simulink library "WECSim_Lib"  (R2014b)
settings: Solver=ode45  StartTime=0.0  StopTime=10.0  RelTol=1e-3
undefined symbols (not defined in the file): body, constraint, pto, simu, waves, X, Y, Z
libraries: nesl_utility x41, sm_lib x35
(part 1 of 2)
settings Model: Creator=cmichel  LastModifiedBy=cmichel

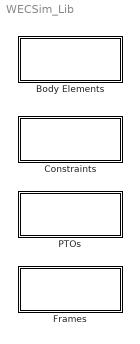
== system WECSim_Lib ==
  Body Elements : Subsystem
      mask Display: text(0,0,' ')
  Constraints : Subsystem
      mask Display: text(0,0,' ')
  Frames : Subsystem
      mask Display: text(0,0,' ')
  PTOs : Subsystem
      mask Display: text(0,0,' ')

== system WECSim_Lib/Body Elements ==
  Rigid Body : Subsystem  mask(BodyElements){body=body(1)}
      mask prompts: body "Body Name:"
      mask help: This block represents a rigid body. The variable name input below must be 'body(i)' where i=1,2,...
      mask init:
      | % Uses:
      | %   body.geometryFile
      | %   body.hydroData.properties.name
      | 
      | if exist('body','var')
      |     h=[gcb '/Structure/Body Properties'];
      |     geomFile=body.geometryFile;
      |     set_param(h,'ExtGeomFileName',geomFile);
      |     h=[gcb '/To Workspace'];
      |     responseName=[body.hydroData.properties.name '_out'];
      |     set_param(h,'VariableName',responseName);
      | end
      | clear bc h geomFile responseName
      settings: AttributesFormatString=%<body>

== system WECSim_Lib/Constraints ==
  Fixed : Subsystem  mask(Constraints){constraint=constraint(1)}
      mask prompts: constraint "Constraint Name:"
      mask help:
      | Does not allow any motion. The variable name input below must be 'constraint(i)' where i=1,2,...
      |
      | constraint(i) must be defined in the input file with the following fields:
      |     .name              = a string
      |     .loc (optional)    = a 3x1 vector [x y z] in m. Default = [0 0 0]
      | The name string is used as the variable name for the output power and as such must comply with all of Matlab's variable naming rules.
      mask init:
      | if exist('constraint','var')
      |     h=[gcb '/output'];
      |     responseName=[constraint.name '_out'];
      |     set_param(h,'VariableName',responseName);
      | end
      | 
      | constraint.checkLoc('W');
      settings: AttributesFormatString=%<constraint>
  Floating : Subsystem  mask(Constraints){constraint=constraint(1)}
      mask prompts: constraint "Constraint Name:"
      mask help:
      | Allows body to be free floating (motion in Surge, Heave, and Pitch). The variable name input below must be 'constraint(i)' where i=1,2,...
      |
      | constraint(i) must be defined in the input file with the following fields:
      |     .name              = a string
      |     .loc (optional)    = a 3x1 vector [x y z] in m. Default = [0 0 0]
      |
      | The name string is used as the variable name for the output power and as such must comply with all of Matlab's variable naming rules.
      mask init:
      | if exist('constraint','var')
      |     h=[gcb '/output'];
      |     responseName=[constraint.name '_out'];
      |     set_param(h,'VariableName',responseName);
      | end
      | 
      | constraint.checkLoc('W');
      settings: AttributesFormatString=%<constraint>
  Heave : Subsystem  mask(Constraints){constraint=constraint(1)}
      mask prompts: constraint "Constraint Name:"
      mask help:
      | Constrains motion to Heave translation only.The variable name input below must be 'constraint(i)' where i=1,2,...
      |
      | constraint(i) must be defined in the input file with the following fields:
      |     .name              = a string
      |     .loc (optional)    = a 3x1 vector [x y z] in m. Default = [0 0 0]
      | The name string is used as the variable name for the output power and as such must comply with all of Matlab's variable naming rules.
      mask init:
      | if exist('constraint','var')
      |     h=[gcb '/output'];
      |     responseName=[constraint.name '_out'];
      |     set_param(h,'VariableName',responseName);
      | end
      | 
      | constraint.checkLoc('W');
      settings: AttributesFormatString=%<constraint>
  Pitch : Subsystem  mask(Constraints){constraint=constraint(1)}
      mask prompts: constraint "Constraint Name:"
      mask help:
      | Constrains motion to Pitch rotation only. The variable name input below must be 'constraint(i)' where i=1,2,...
      |
      | constraint(i) must be defined in the input file with the following fields:
      |     .name   = a string
      |     .loc    = a 3x1 vector [x y z] in m
      |
      | The name string is used as the variable name for the output power and as such must comply with all of Matlab's variable naming rules.
      mask init:
      | if exist('constraint','var')
      |     h=[gcb '/output'];
      |     responseName=[constraint.name '_out'];
      |     set_param(h,'VariableName',responseName);
      | end
      | 
      | constraint.checkLoc('E');
      settings: AttributesFormatString=%<constraint>
  Surge : Subsystem  mask(Constraints){constraint=constraint(1)}
      mask prompts: constraint "Constraint Name:"
      mask help:
      | Constrains motion to Surge translation only.The variable name input below must be 'constraint(i)' where i=1,2,...
      |
      | constraint(i) must be defined in the input file with the following fields:
      |     .name              = a string
      |     .loc (optional)    = a 3x1 vector [x y z] in m. Default = [0 0 0]
      |
      | The name string is used as the variable name for the output power and as such must comply with all of Matlab's variable naming rules.
      mask init:
      | if exist('constraint','var')
      |     h=[gcb '/output'];
      |     responseName=[constraint.name '_out'];
      |     set_param(h,'VariableName',responseName);
      | end
      | 
      | constraint.checkLoc('W');
      settings: AttributesFormatString=%<constraint>

== system WECSim_Lib/Frames ==
  Global Reference Frame : Subsystem  mask(Frames){waves=waves, simu=simu}
      mask prompts: waves "Wave Class Name"; simu "Simulation Class Name"
      mask help:
      | This block contains Global References, including solver configurations, free surface and seabed description, and simulation time.
      | It uses the following fields from the Simulation and Wave classes:
      |
      | Simulation Class:
      |     .endTime
      |     .dt
      |     .domainSize
      |
      | Wave Class:
      |     .waterDepth

== system WECSim_Lib/PTOs ==
  Rotational PTO (Local RY) : Subsystem  mask(PTO){pto=pto(1)}
      mask prompts: pto "PTO Name:"
      mask help:
      | This PTO constrains the follower (F) to only rotate about the Y-axis of the base (B), and applies a PTO stiffness and damping value. The variable name input below must be 'pto(i)' where i=1,2,...
      |
      | pto(i) must be defined in the input file with the following fields:
      |     .name   = a string
      |     .k      = a scalar in N*m/radians
      |     .c      = a scalar in N*m/(radians/s)
      |     .loc    = a 3x1 vector [x y z] in m
      |
      | The name string is used as the variable name for the output power and as such must comply with all of Matlab's variable naming rules.
      mask init:
      | if exist('pto','var')
      |     h=[gcb '/output'];
      |     responseName=[pto.name '_out'];
      |     set_param(h,'VariableName',responseName);
      | end
      | 
      | pto.checkLoc('E');
      settings: AttributesFormatString=%<pto>
  Translational PTO (Local X) : Subsystem  mask(PTO){pto=pto(1)}
      mask prompts: pto "PTO Name:"
      mask help:
      | This PTO constrains the follower (F) to only move along the X-direction of the base (B), and applies a PTO stiffness and damping value. The variable name input below must be 'pto(i)' where i=1,2,...
      |
      | pto(i) must be defined in the input file with the following fields:
      |     .name              = a string
      |     .k                 = a scalar in N/m
      |     .c                 = a scalar in N/(m/s)
      |     .loc (optional)    = a 3x1 vector [x y z] in m. Default = [0 0 0]
      | The name string is used as the variable name for the output power and as such must comply with all of Matlab's variable naming rules.
      mask init:
      | if exist('pto','var')
      |     h=[gcb '/output'];
      |     responseName=[pto.name '_out'];
      |     set_param(h,'VariableName',responseName);
      | end
      | 
      | pto.checkLoc('W');
      settings: AttributesFormatString=%<pto>
  Translational PTO (Local Z) : Subsystem  mask(PTO){pto=pto(1)}
      mask prompts: pto "PTO Name:"
      mask help:
      | This PTO constrains the follower (F) to only move along the Z-direction of the base (B), and applies a PTO stiffness and damping value. The variable name input below must be 'pto(i)' where i=1,2,...
      |
      | pto(i) must be defined in the input file with the following fields:
      |     .name               = a string
      |     .k                  = a scalar in N/m
      |     .c                  = a scalar in N/(m/s)
      |     .loc (optional)     = a 3x1 vector [x y z] in m. Default = [0 0 0]
      |
      | The name string is used as the variable name for the output power and as such must comply with all of Matlab's variable naming rules.
      mask init:
      | if exist('pto','var')
      |     h=[gcb '/output'];
      |     responseName=[pto.name '_out'];
      |     set_param(h,'VariableName',responseName);
      | end
      | 
      | pto.checkLoc('W');
      settings: AttributesFormatString=%<pto>

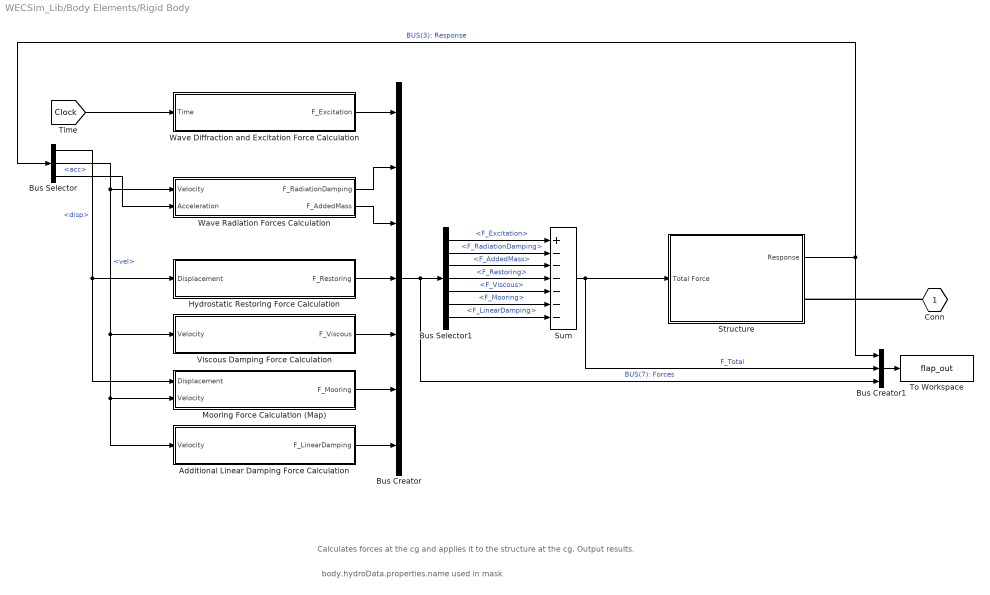
== system WECSim_Lib/Body Elements/Rigid Body ==
  note: body.hydroData.properties.name used in mask
  note: Calculates forces at the cg and applies it to the structure at the cg. Output results.
  Additional Linear Damping Force Calculation : Subsystem
  Bus Creator : BusCreator  Inputs=7
  Bus Creator1 : BusCreator  Inputs=3
  Bus Selector : BusSelector  OutputSignals=disp,vel,acc
  Bus Selector1 : BusSelector  OutputSignals=F_Excitation,F_RadiationDamping,F_AddedMass,F_Restoring,F_Viscous,F_Mooring,F_LinearDamping
  Hydrostatic Restoring Force Calculation : Subsystem
  Mooring Force Calculation (Map) : Subsystem
  Structure : Subsystem
  Sum : Sum  Inputs=+------
  To Workspace : ToWorkspace  VariableName=flap_out  SaveFormat=Structure With Time  SampleTime=-1
  Viscous Damping Force Calculation : Subsystem
  Wave Diffraction and Excitation Force Calculation : Subsystem
  Wave Radiation Forces Calculation : Subsystem
  Conn : PMIOPort  Port=1  Side=Right
  wires:
  Sum/1 -> Bus Creator1/2, Structure/1(Total Force)  "F_Total"
  Bus Selector/1 -> Mooring Force Calculation (Map)/1(Displacement), Hydrostatic Restoring Force Calculation/1(Displacement)  "<disp>"
  Structure/1(Response) -> Bus Creator1/1, Bus Selector/1  "BUS(3): Response"
  Bus Creator/1 -> Bus Creator1/3, Bus Selector1/1  "BUS(7): Forces"
  Bus Creator1/1 -> To Workspace/1
  Mooring Force Calculation (Map)/1(F_Mooring) -> Bus Creator/6
  Viscous Damping Force Calculation/1(F_Viscous) -> Bus Creator/5
  Hydrostatic Restoring Force Calculation/1(F_Restoring) -> Bus Creator/4
  Wave Radiation Forces Calculation/1(F_RadiationDamping) -> Bus Creator/2
  Wave Diffraction and Excitation Force Calculation/1(F_Excitation) -> Bus Creator/1
  Additional Linear Damping Force Calculation/1(F_LinearDamping) -> Bus Creator/7
  Bus Selector/2 -> Additional Linear Damping Force Calculation/1(Velocity), Mooring Force Calculation (Map)/2(Velocity), Viscous Damping Force Calculation/1(Velocity), Wave Radiation Forces Calculation/1(Velocity)  "<vel>"
  Bus Selector/3 -> Wave Radiation Forces Calculation/2(Acceleration)  "<acc>"
  Wave Radiation Forces Calculation/2(F_AddedMass) -> Bus Creator/3
  Bus Selector1/4 -> Sum/4  "<F_Restoring>"
  Bus Selector1/3 -> Sum/3  "<F_AddedMass>"
  Bus Selector1/5 -> Sum/5  "<F_Viscous>"
  Bus Selector1/2 -> Sum/2  "<F_RadiationDamping>"
  Bus Selector1/6 -> Sum/6  "<F_Mooring>"
  Bus Selector1/1 -> Sum/1  "<F_Excitation>"
  Bus Selector1/7 -> Sum/7  "<F_LinearDamping>"
  [Clock] -> Wave Diffraction and Excitation Force Calculation/1(Time)
  connections:
  Conn/RConn1 -- Structure/RConn1

== system WECSim_Lib/Constraints/Fixed ==
  note: constraint.loc
      | constraint.c
      | constraint.k
      | constraint.name used in mask
  note: Constraints the motion to the desired DOF.
      | Moves the connection points (B and F) from the free surface to the PTO location.
      | Outputs forces and motions.
  Mux : Mux  Inputs=2
  PS-Simulink Converter : nesl_utility/PS-Simulink Converter  PhysicalDomain=network_engine_domain  SubClassName=ps_output  LeftPortType=input  RightPortType=output  PseudoPeriodic=off  Frequencies=[]  Unit=1  AffineConversion=off
  PS-Simulink Converter1 : nesl_utility/PS-Simulink Converter  PhysicalDomain=network_engine_domain  SubClassName=ps_output  LeftPortType=input  RightPortType=output  PseudoPeriodic=off  Frequencies=[]  Unit=1  AffineConversion=off
  Rigid Transform : sm_lib/Frames and Transforms/Rigid Transform  TranslationMethod=Cartesian  TranslationLengthUnit=m  TranslationStandardAxis=+Z  TranslationStandardOffset=0  TranslationCartesianOffset=constraint.loc  TranslationROffset=0  TranslationROffsetUnits=m  TranslationZOffset=0  TranslationZOffsetUnits=m  TranslationThetaOffset=0  TranslationThetaOffsetUnits=deg  RotationMethod=None  RotationAngleUnits=deg  RotationStandardAxis=+X  RotationAngle=90  RotationArbitraryAxis=[0 0 1]  FollAlignAxisA=+X  BaseAlignAxisA=+Y  FollAlignAxisB=+Y  BaseAlignAxisB=+Z  RotationMatrix=[1 0 0; 0 1 0; 0 0 1]  BlockFunction=simmechanics.library.frames_transforms.rigid_transform
  Rigid Transform1 : sm_lib/Frames and Transforms/Rigid Transform  TranslationMethod=Cartesian  TranslationLengthUnit=m  TranslationStandardAxis=+Z  TranslationStandardOffset=0  TranslationCartesianOffset=constraint.loc  TranslationROffset=0  TranslationROffsetUnits=m  TranslationZOffset=0  TranslationZOffsetUnits=m  TranslationThetaOffset=0  TranslationThetaOffsetUnits=deg  RotationMethod=None  RotationAngleUnits=deg  RotationStandardAxis=+X  RotationAngle=90  RotationArbitraryAxis=[0 0 1]  FollAlignAxisA=+X  BaseAlignAxisA=+Y  FollAlignAxisB=+Y  BaseAlignAxisB=+Z  RotationMatrix=[1 0 0; 0 1 0; 0 0 1]  BlockFunction=simmechanics.library.frames_transforms.rigid_transform
  Weld Joint (Fixed) : sm_lib/Joints/Weld Joint  SenseConstraintForce=on  SenseConstraintForceX=off  SenseConstraintForceY=off  SenseConstraintForceZ=off  SenseConstraintTorque=on  SenseConstraintTorqueX=off  SenseConstraintTorqueY=off  SenseConstraintTorqueZ=off  SenseTotalForce=off  SenseTotalForceX=off  SenseTotalForceY=off  SenseTotalForceZ=off  SenseTotalTorque=off  SenseTotalTorqueX=off  SenseTotalTorqueY=off  SenseTotalTorqueZ=off  CompositeWrenchDir=BaseOnFollower  CompositeWrenchFrame=BaseFrame  BlockFunction=simmechanics.library.joints.weld_joint
  output : ToWorkspace  VariableName=Constraint1_out  SaveFormat=Structure With Time  SampleTime=-1
  B : PMIOPort  Port=1  Side=Left
  F : PMIOPort  Port=2  Side=Right
  wires:
  PS-Simulink Converter/1 -> Mux/1
  PS-Simulink Converter1/1 -> Mux/2
  Mux/1 -> output/1  "Constraint Forces"
  connections:
  PS-Simulink Converter1/LConn1 -- Weld Joint (Fixed)/RConn3
  PS-Simulink Converter/LConn1 -- Weld Joint (Fixed)/RConn2
  F/RConn1 -- Rigid Transform1/LConn1
  Rigid Transform1/RConn1 -- Weld Joint (Fixed)/RConn1
  Weld Joint (Fixed)/LConn1 -- Rigid Transform/RConn1
  Rigid Transform/LConn1 -- B/RConn1

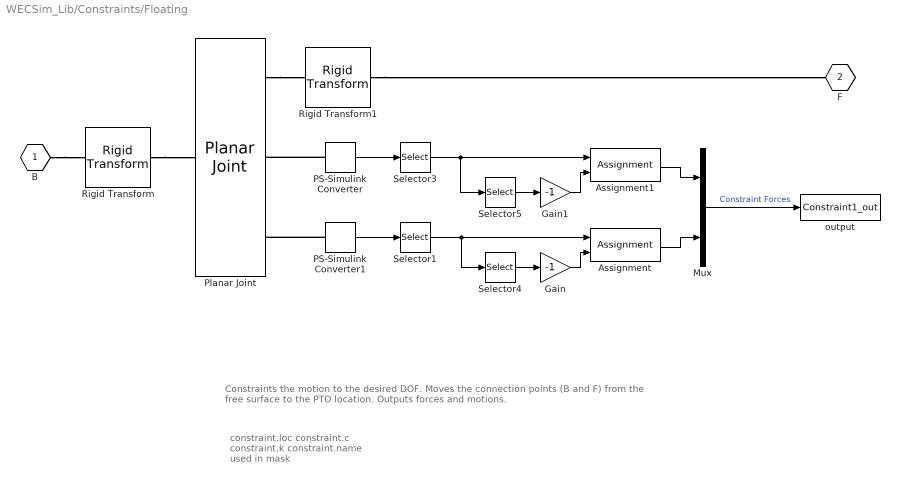
== system WECSim_Lib/Constraints/Floating ==
  note: constraint.loc
      | constraint.c
      | constraint.k
      | constraint.name used in mask
  note: Constraints the motion to the desired DOF.
      | Moves the connection points (B and F) from the free surface to the PTO location.
      | Outputs forces and motions.
  Assignment : Assignment  DiagnosticForDimensions=Warning  Indices=2
  Assignment1 : Assignment  DiagnosticForDimensions=Warning  Indices=2
  Gain : Gain  Gain=-1
  Gain1 : Gain  Gain=-1
  Mux : Mux  Inputs=2
  PS-Simulink Converter : nesl_utility/PS-Simulink Converter  PhysicalDomain=network_engine_domain  SubClassName=ps_output  LeftPortType=input  RightPortType=output  PseudoPeriodic=off  Frequencies=[]  Unit=1  AffineConversion=off
  PS-Simulink Converter1 : nesl_utility/PS-Simulink Converter  PhysicalDomain=network_engine_domain  SubClassName=ps_output  LeftPortType=input  RightPortType=output  PseudoPeriodic=off  Frequencies=[]  Unit=1  AffineConversion=off
  Planar Joint : sm_lib/Joints/Planar Joint  SenseConstraintForce=on  SenseConstraintForceX=off  SenseConstraintForceY=off  SenseConstraintForceZ=off  SenseConstraintTorque=on  SenseConstraintTorqueX=off  SenseConstraintTorqueY=off  SenseConstraintTorqueZ=off  SenseTotalForce=off  SenseTotalForceX=off  SenseTotalForceY=off  SenseTotalForceZ=off  SenseTotalTorque=off  SenseTotalTorqueX=off  SenseTotalTorqueY=off  SenseTotalTorqueZ=off  CompositeWrenchDir=BaseOnFollower  CompositeWrenchFrame=BaseFrame  PxEquilibriumPosition=0  PxEquilibriumPositionUnits=m  PxSpringStiffness=0  PxSpringStiffnessUnits=N/m  PxDampingCoefficient=0  PxDampingCoefficientUnits=N/(m/s)  PxTorqueActuationMode=NoTorque  PxMotionActuationMode=ComputedMotion  PxSensePosition=off  PxSenseVelocity=off  PxSenseAcceleration=off  PxSenseTorqueForce=off  PxPositionTargetValue=0  PxPositionTargetValueUnits=m  PxPositionTargetSpecify=off  PxPositionTargetPriority=High  PxVelocityTargetValue=0  PxVelocityTargetValueUnits=m/s  PxVelocityTargetSpecify=off  PxVelocityTargetPriority=High  PyEquilibriumPosition=0  PyEquilibriumPositionUnits=m  PySpringStiffness=0  PySpringStiffnessUnits=N/m  PyDampingCoefficient=0  PyDampingCoefficientUnits=N/(m/s)  PyTorqueActuationMode=NoTorque  PyMotionActuationMode=ComputedMotion  PySensePosition=off  PySenseVelocity=off  PySenseAcceleration=off  PySenseTorqueForce=off  PyPositionTargetValue=0  PyPositionTargetValueUnits=m  PyPositionTargetSpecify=off  PyPositionTargetPriority=High  PyVelocityTargetValue=0  PyVelocityTargetValueUnits=m/s  PyVelocityTargetSpecify=off  PyVelocityTargetPriority=High  RzEquilibriumPosition=0  RzEquilibriumPositionUnits=deg  RzSpringStiffness=0  RzSpringStiffnessUnits=N*m/deg  RzDampingCoefficient=0  RzDampingCoefficientUnits=N*m/(deg/s)  RzTorqueActuationMode=NoTorque  RzMotionActuationMode=ComputedMotion  RzSensePosition=off  RzSenseVelocity=off  RzSenseAcceleration=off  RzSenseTorqueForce=off  RzPositionTargetValue=0  RzPositionTargetValueUnits=deg  RzPositionTargetSpecify=off  RzPositionTargetPriority=High  RzVelocityTargetValue=0  RzVelocityTargetValueUnits=deg/s  RzVelocityTargetSpecify=off  RzVelocityTargetPriority=High  BlockFunction=simmechanics.library.joints.planar_joint
  Rigid Transform : sm_lib/Frames and Transforms/Rigid Transform  TranslationMethod=Cartesian  TranslationLengthUnit=m  TranslationStandardAxis=+Z  TranslationStandardOffset=0  TranslationCartesianOffset=constraint.loc  TranslationROffset=0  TranslationROffsetUnits=m  TranslationZOffset=0  TranslationZOffsetUnits=m  TranslationThetaOffset=0  TranslationThetaOffsetUnits=deg  RotationMethod=StandardAxis  RotationAngleUnits=deg  RotationStandardAxis=+X  RotationAngle=90  RotationArbitraryAxis=[0 0 1]  FollAlignAxisA=+X  BaseAlignAxisA=+Y  FollAlignAxisB=+Y  BaseAlignAxisB=+Z  RotationMatrix=[1 0 0; 0 1 0; 0 0 1]  BlockFunction=simmechanics.library.frames_transforms.rigid_transform
  Rigid Transform1 : sm_lib/Frames and Transforms/Rigid Transform  TranslationMethod=Cartesian  TranslationLengthUnit=m  TranslationStandardAxis=+Z  TranslationStandardOffset=0  TranslationCartesianOffset=constraint.loc  TranslationROffset=0  TranslationROffsetUnits=m  TranslationZOffset=0  TranslationZOffsetUnits=m  TranslationThetaOffset=0  TranslationThetaOffsetUnits=deg  RotationMethod=StandardAxis  RotationAngleUnits=deg  RotationStandardAxis=+X  RotationAngle=90  RotationArbitraryAxis=[0 0 1]  FollAlignAxisA=+X  BaseAlignAxisA=+Y  FollAlignAxisB=+Y  BaseAlignAxisB=+Z  RotationMatrix=[1 0 0; 0 1 0; 0 0 1]  BlockFunction=simmechanics.library.frames_transforms.rigid_transform
  Selector1 : Selector  InputPortWidth=3  Indices=[1 3 2]
  Selector3 : Selector  InputPortWidth=3  Indices=[1 3 2]
  Selector4 : Selector  InputPortWidth=3  Indices=[2]
  Selector5 : Selector  InputPortWidth=3  Indices=[2]
  output : ToWorkspace  VariableName=Constraint1_out  SaveFormat=Structure With Time  SampleTime=-1
  B : PMIOPort  Port=1  Side=Left
  F : PMIOPort  Port=2  Side=Right
  wires:
  Mux/1 -> output/1  "Constraint Forces"
  Selector1/1 -> Assignment/1, Selector4/1
  Selector4/1 -> Gain/1
  Gain/1 -> Assignment/2
  Selector3/1 -> Assignment1/1, Selector5/1
  Selector5/1 -> Gain1/1
  Gain1/1 -> Assignment1/2
  PS-Simulink Converter1/1 -> Selector1/1
  PS-Simulink Converter/1 -> Selector3/1
  Assignment/1 -> Mux/2
  Assignment1/1 -> Mux/1
  connections:
  Rigid Transform1/LConn1 -- F/RConn1
  Planar Joint/RConn1 -- Rigid Transform1/RConn1
  Rigid Transform/RConn1 -- Planar Joint/LConn1
  B/RConn1 -- Rigid Transform/LConn1
  PS-Simulink Converter/LConn1 -- Planar Joint/RConn2
  PS-Simulink Converter1/LConn1 -- Planar Joint/RConn3

== system WECSim_Lib/Constraints/Heave ==
  note: constraint.loc
      | constraint.c
      | constraint.k
      | constraint.name used in mask
  note: Constraints the motion to the desired DOF.
      | Moves the connection points (B and F) from the free surface to the PTO location.
      | Outputs forces and motions.
  Mux : Mux  Inputs=2
  PS-Simulink Converter : nesl_utility/PS-Simulink Converter  PhysicalDomain=network_engine_domain  SubClassName=ps_output  LeftPortType=input  RightPortType=output  PseudoPeriodic=off  Frequencies=[]  Unit=1  AffineConversion=off
  PS-Simulink Converter1 : nesl_utility/PS-Simulink Converter  PhysicalDomain=network_engine_domain  SubClassName=ps_output  LeftPortType=input  RightPortType=output  PseudoPeriodic=off  Frequencies=[]  Unit=1  AffineConversion=off
  Prismatic Joint (Translational Constraint) : sm_lib/Joints/Prismatic Joint  SenseConstraintForce=on  SenseConstraintForceX=off  SenseConstraintForceY=off  SenseConstraintForceZ=off  SenseConstraintTorque=on  SenseConstraintTorqueX=off  SenseConstraintTorqueY=off  SenseConstraintTorqueZ=off  SenseTotalForce=off  SenseTotalForceX=off  SenseTotalForceY=off  SenseTotalForceZ=off  SenseTotalTorque=off  SenseTotalTorqueX=off  SenseTotalTorqueY=off  SenseTotalTorqueZ=off  CompositeWrenchDir=BaseOnFollower  CompositeWrenchFrame=BaseFrame  EquilibriumPosition=0  EquilibriumPositionUnits=m  SpringStiffness=0  SpringStiffnessUnits=N/m  DampingCoefficient=0  DampingCoefficientUnits=N/(m/s)  TorqueActuationMode=NoTorque  MotionActuationMode=ComputedMotion  SensePosition=off  SenseVelocity=off  SenseAcceleration=off  SenseTorqueForce=off  PositionTargetValue=0  PositionTargetValueUnits=m  PositionTargetSpecify=off  PositionTargetPriority=High  VelocityTargetValue=0  VelocityTargetValueUnits=m/s  VelocityTargetSpecify=off  VelocityTargetPriority=High  BlockFunction=simmechanics.library.joints.prismatic_joint
  Rigid Transform : sm_lib/Frames and Transforms/Rigid Transform  TranslationMethod=Cartesian  TranslationLengthUnit=m  TranslationStandardAxis=+Z  TranslationStandardOffset=0  TranslationCartesianOffset=constraint.loc  TranslationROffset=0  TranslationROffsetUnits=m  TranslationZOffset=0  TranslationZOffsetUnits=m  TranslationThetaOffset=0  TranslationThetaOffsetUnits=deg  RotationMethod=None  RotationAngleUnits=deg  RotationStandardAxis=+X  RotationAngle=90  RotationArbitraryAxis=[0 0 1]  FollAlignAxisA=+X  BaseAlignAxisA=+Y  FollAlignAxisB=+Y  BaseAlignAxisB=+Z  RotationMatrix=[1 0 0; 0 1 0; 0 0 1]  BlockFunction=simmechanics.library.frames_transforms.rigid_transform
  Rigid Transform1 : sm_lib/Frames and Transforms/Rigid Transform  TranslationMethod=Cartesian  TranslationLengthUnit=m  TranslationStandardAxis=+Z  TranslationStandardOffset=0  TranslationCartesianOffset=constraint.loc  TranslationROffset=0  TranslationROffsetUnits=m  TranslationZOffset=0  TranslationZOffsetUnits=m  TranslationThetaOffset=0  TranslationThetaOffsetUnits=deg  RotationMethod=None  RotationAngleUnits=deg  RotationStandardAxis=+X  RotationAngle=90  RotationArbitraryAxis=[0 0 1]  FollAlignAxisA=+X  BaseAlignAxisA=+Y  FollAlignAxisB=+Y  BaseAlignAxisB=+Z  RotationMatrix=[1 0 0; 0 1 0; 0 0 1]  BlockFunction=simmechanics.library.frames_transforms.rigid_transform
  output : ToWorkspace  VariableName=Constraint1_out  SaveFormat=Structure With Time  SampleTime=-1
  F : PMIOPort  Port=1  Side=Right
  B : PMIOPort  Port=2  Side=Left
  wires:
  PS-Simulink Converter/1 -> Mux/1
  PS-Simulink Converter1/1 -> Mux/2
  Mux/1 -> output/1  "Constraint Forces"
  connections:
  PS-Simulink Converter/LConn1 -- Prismatic Joint (Translational Constraint)/RConn2
  PS-Simulink Converter1/LConn1 -- Prismatic Joint (Translational Constraint)/RConn3
  Rigid Transform1/RConn1 -- Prismatic Joint (Translational Constraint)/RConn1
  Rigid Transform1/LConn1 -- F/RConn1
  B/RConn1 -- Rigid Transform/LConn1
  Rigid Transform/RConn1 -- Prismatic Joint (Translational Constraint)/LConn1

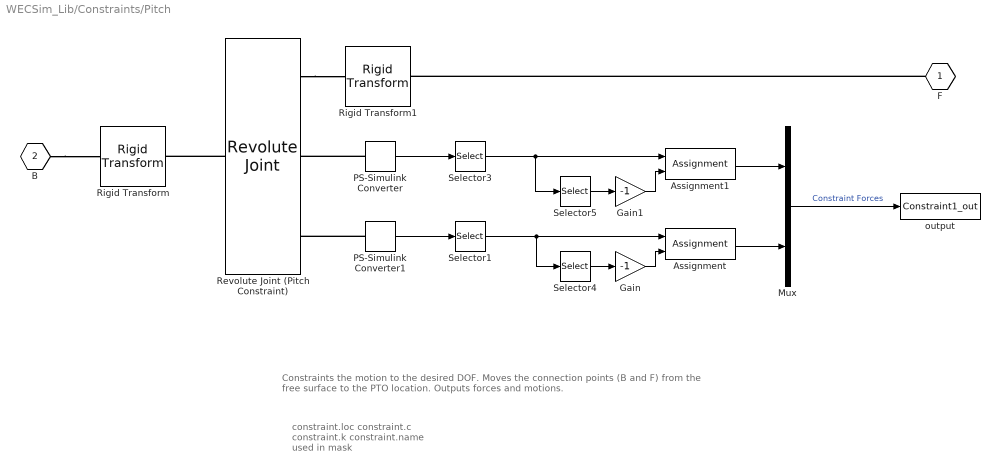
== system WECSim_Lib/Constraints/Pitch ==
  note: constraint.loc
      | constraint.c
      | constraint.k
      | constraint.name used in mask
  note: Constraints the motion to the desired DOF.
      | Moves the connection points (B and F) from the free surface to the PTO location.
      | Outputs forces and motions.
  Assignment : Assignment  DiagnosticForDimensions=Warning  Indices=2
  Assignment1 : Assignment  DiagnosticForDimensions=Warning  Indices=2
  Gain : Gain  Gain=-1
  Gain1 : Gain  Gain=-1
  Mux : Mux  Inputs=2
  PS-Simulink Converter : nesl_utility/PS-Simulink Converter  PhysicalDomain=network_engine_domain  SubClassName=ps_output  LeftPortType=input  RightPortType=output  PseudoPeriodic=off  Frequencies=[]  Unit=1  AffineConversion=off
  PS-Simulink Converter1 : nesl_utility/PS-Simulink Converter  PhysicalDomain=network_engine_domain  SubClassName=ps_output  LeftPortType=input  RightPortType=output  PseudoPeriodic=off  Frequencies=[]  Unit=1  AffineConversion=off
  Revolute Joint (Pitch Constraint) : sm_lib/Joints/Revolute Joint  SenseConstraintForce=on  SenseConstraintForceX=off  SenseConstraintForceY=off  SenseConstraintForceZ=off  SenseConstraintTorque=on  SenseConstraintTorqueX=off  SenseConstraintTorqueY=off  SenseConstraintTorqueZ=off  SenseTotalForce=off  SenseTotalForceX=off  SenseTotalForceY=off  SenseTotalForceZ=off  SenseTotalTorque=off  SenseTotalTorqueX=off  SenseTotalTorqueY=off  SenseTotalTorqueZ=off  CompositeWrenchDir=BaseOnFollower  CompositeWrenchFrame=BaseFrame  EquilibriumPosition=0  EquilibriumPositionUnits=deg  SpringStiffness=0  SpringStiffnessUnits=N*m/deg  DampingCoefficient=0  DampingCoefficientUnits=N*m/(rad/s)  TorqueActuationMode=NoTorque  MotionActuationMode=ComputedMotion  SensePosition=off  SenseVelocity=off  SenseAcceleration=off  SenseTorqueForce=off  PositionTargetValue=0  PositionTargetValueUnits=deg  PositionTargetSpecify=off  PositionTargetPriority=High  VelocityTargetValue=0  VelocityTargetValueUnits=deg/s  VelocityTargetSpecify=off  VelocityTargetPriority=High  BlockFunction=simmechanics.library.joints.revolute_joint
  Rigid Transform : sm_lib/Frames and Transforms/Rigid Transform  TranslationMethod=Cartesian  TranslationLengthUnit=m  TranslationStandardAxis=+Z  TranslationStandardOffset=0  TranslationCartesianOffset=constraint.loc  TranslationROffset=0  TranslationROffsetUnits=m  TranslationZOffset=0  TranslationZOffsetUnits=m  TranslationThetaOffset=0  TranslationThetaOffsetUnits=deg  RotationMethod=StandardAxis  RotationAngleUnits=deg  RotationStandardAxis=+X  RotationAngle=90  RotationArbitraryAxis=[0 0 1]  FollAlignAxisA=+X  BaseAlignAxisA=+Y  FollAlignAxisB=+Y  BaseAlignAxisB=+Z  RotationMatrix=[1 0 0; 0 1 0; 0 0 1]  BlockFunction=simmechanics.library.frames_transforms.rigid_transform
  Rigid Transform1 : sm_lib/Frames and Transforms/Rigid Transform  TranslationMethod=Cartesian  TranslationLengthUnit=m  TranslationStandardAxis=+Z  TranslationStandardOffset=0  TranslationCartesianOffset=constraint.loc  TranslationROffset=0  TranslationROffsetUnits=m  TranslationZOffset=0  TranslationZOffsetUnits=m  TranslationThetaOffset=0  TranslationThetaOffsetUnits=deg  RotationMethod=StandardAxis  RotationAngleUnits=deg  RotationStandardAxis=+X  RotationAngle=90  RotationArbitraryAxis=[0 0 1]  FollAlignAxisA=+X  BaseAlignAxisA=+Y  FollAlignAxisB=+Y  BaseAlignAxisB=+Z  RotationMatrix=[1 0 0; 0 1 0; 0 0 1]  BlockFunction=simmechanics.library.frames_transforms.rigid_transform
  Selector1 : Selector  InputPortWidth=3  Indices=[1 3 2]
  Selector3 : Selector  InputPortWidth=3  Indices=[1 3 2]
  Selector4 : Selector  InputPortWidth=3  Indices=[2]
  Selector5 : Selector  InputPortWidth=3  Indices=[2]
  output : ToWorkspace  VariableName=Constraint1_out  SaveFormat=Structure With Time  SampleTime=-1
  F : PMIOPort  Port=1  Side=Right
  B : PMIOPort  Port=2  Side=Left
  wires:
  Mux/1 -> output/1  "Constraint Forces"
  PS-Simulink Converter/1 -> Selector3/1
  PS-Simulink Converter1/1 -> Selector1/1
  Selector1/1 -> Selector4/1, Assignment/1
  Selector4/1 -> Gain/1
  Gain/1 -> Assignment/2
  Assignment/1 -> Mux/2
  Selector3/1 -> Selector5/1, Assignment1/1
  Selector5/1 -> Gain1/1
  Gain1/1 -> Assignment1/2
  Assignment1/1 -> Mux/1
  connections:
  Revolute Joint (Pitch Constraint)/LConn1 -- Rigid Transform/RConn1
  Revolute Joint (Pitch Constraint)/RConn1 -- Rigid Transform1/RConn1
  B/RConn1 -- Rigid Transform/LConn1
  F/RConn1 -- Rigid Transform1/LConn1
  PS-Simulink Converter/LConn1 -- Revolute Joint (Pitch Constraint)/RConn2
  PS-Simulink Converter1/LConn1 -- Revolute Joint (Pitch Constraint)/RConn3

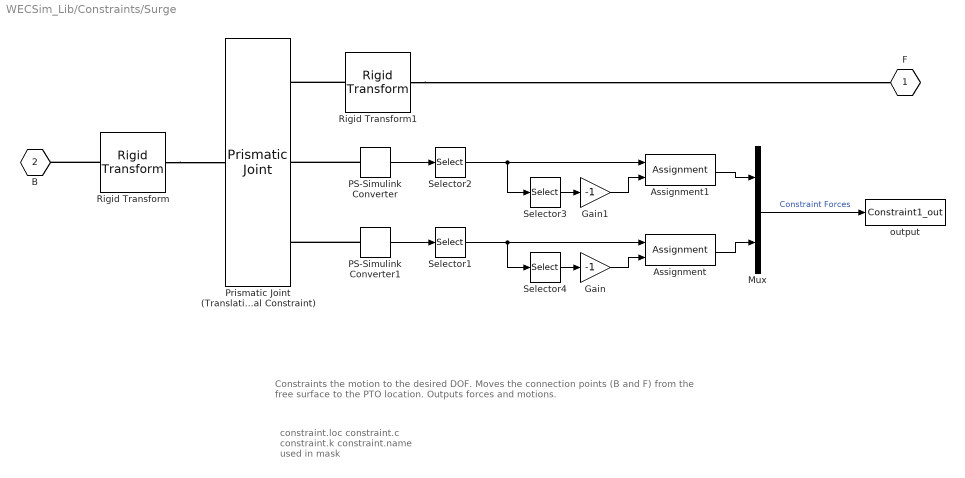
== system WECSim_Lib/Constraints/Surge ==
  note: constraint.loc
      | constraint.c
      | constraint.k
      | constraint.name used in mask
  note: Constraints the motion to the desired DOF.
      | Moves the connection points (B and F) from the free surface to the PTO location.
      | Outputs forces and motions.
  Assignment : Assignment  DiagnosticForDimensions=Warning  Indices=3
  Assignment1 : Assignment  DiagnosticForDimensions=Warning  Indices=3
  Gain : Gain  Gain=-1
  Gain1 : Gain  Gain=-1
  Mux : Mux  Inputs=2
  PS-Simulink Converter : nesl_utility/PS-Simulink Converter  PhysicalDomain=network_engine_domain  SubClassName=ps_output  LeftPortType=input  RightPortType=output  PseudoPeriodic=off  Frequencies=[]  Unit=1  AffineConversion=off
  PS-Simulink Converter1 : nesl_utility/PS-Simulink Converter  PhysicalDomain=network_engine_domain  SubClassName=ps_output  LeftPortType=input  RightPortType=output  PseudoPeriodic=off  Frequencies=[]  Unit=1  AffineConversion=off
  Prismatic Joint (Translational Constraint) : sm_lib/Joints/Prismatic Joint  SenseConstraintForce=on  SenseConstraintForceX=off  SenseConstraintForceY=off  SenseConstraintForceZ=off  SenseConstraintTorque=on  SenseConstraintTorqueX=off  SenseConstraintTorqueY=off  SenseConstraintTorqueZ=off  SenseTotalForce=off  SenseTotalForceX=off  SenseTotalForceY=off  SenseTotalForceZ=off  SenseTotalTorque=off  SenseTotalTorqueX=off  SenseTotalTorqueY=off  SenseTotalTorqueZ=off  CompositeWrenchDir=BaseOnFollower  CompositeWrenchFrame=BaseFrame  EquilibriumPosition=0  EquilibriumPositionUnits=m  SpringStiffness=0  SpringStiffnessUnits=N/m  DampingCoefficient=0  DampingCoefficientUnits=N/(m/s)  TorqueActuationMode=NoTorque  MotionActuationMode=ComputedMotion  SensePosition=off  SenseVelocity=off  SenseAcceleration=off  SenseTorqueForce=off  PositionTargetValue=0  PositionTargetValueUnits=m  PositionTargetSpecify=off  PositionTargetPriority=High  VelocityTargetValue=0  VelocityTargetValueUnits=m/s  VelocityTargetSpecify=off  VelocityTargetPriority=High  BlockFunction=simmechanics.library.joints.prismatic_joint
  Rigid Transform : sm_lib/Frames and Transforms/Rigid Transform  TranslationMethod=Cartesian  TranslationLengthUnit=m  TranslationStandardAxis=+Z  TranslationStandardOffset=0  TranslationCartesianOffset=constraint.loc  TranslationROffset=0  TranslationROffsetUnits=m  TranslationZOffset=0  TranslationZOffsetUnits=m  TranslationThetaOffset=0  TranslationThetaOffsetUnits=deg  RotationMethod=StandardAxis  RotationAngleUnits=deg  RotationStandardAxis=+Y  RotationAngle=90  RotationArbitraryAxis=[0 0 1]  FollAlignAxisA=+X  BaseAlignAxisA=+Y  FollAlignAxisB=+Y  BaseAlignAxisB=+Z  RotationMatrix=[1 0 0; 0 1 0; 0 0 1]  BlockFunction=simmechanics.library.frames_transforms.rigid_transform
  Rigid Transform1 : sm_lib/Frames and Transforms/Rigid Transform  TranslationMethod=Cartesian  TranslationLengthUnit=m  TranslationStandardAxis=+Z  TranslationStandardOffset=0  TranslationCartesianOffset=constraint.loc  TranslationROffset=0  TranslationROffsetUnits=m  TranslationZOffset=0  TranslationZOffsetUnits=m  TranslationThetaOffset=0  TranslationThetaOffsetUnits=deg  RotationMethod=StandardAxis  RotationAngleUnits=deg  RotationStandardAxis=+Y  RotationAngle=90  RotationArbitraryAxis=[0 0 1]  FollAlignAxisA=+X  BaseAlignAxisA=+Y  FollAlignAxisB=+Y  BaseAlignAxisB=+Z  RotationMatrix=[1 0 0; 0 1 0; 0 0 1]  BlockFunction=simmechanics.library.frames_transforms.rigid_transform
  Selector1 : Selector  InputPortWidth=3  Indices=[3 2 1]
  Selector2 : Selector  InputPortWidth=3  Indices=[3 2 1]
  Selector3 : Selector  InputPortWidth=3  Indices=[3]
  Selector4 : Selector  InputPortWidth=3  Indices=[3]
  output : ToWorkspace  VariableName=Constraint1_out  SaveFormat=Structure With Time  SampleTime=-1
  F : PMIOPort  Port=1  Side=Right
  B : PMIOPort  Port=2  Side=Left
  wires:
  Mux/1 -> output/1  "Constraint Forces"
  Selector1/1 -> Selector4/1, Assignment/1
  Selector4/1 -> Gain/1
  Gain/1 -> Assignment/2
  Selector2/1 -> Selector3/1, Assignment1/1
  Selector3/1 -> Gain1/1
  Gain1/1 -> Assignment1/2
  Assignment/1 -> Mux/2
  Assignment1/1 -> Mux/1
  PS-Simulink Converter1/1 -> Selector1/1
  PS-Simulink Converter/1 -> Selector2/1
  connections:
  Rigid Transform1/LConn1 -- F/RConn1
  Rigid Transform1/RConn1 -- Prismatic Joint (Translational Constraint)/RConn1
  Rigid Transform/RConn1 -- Prismatic Joint (Translational Constraint)/LConn1
  Rigid Transform/LConn1 -- B/RConn1
  PS-Simulink Converter/LConn1 -- Prismatic Joint (Translational Constraint)/RConn2
  PS-Simulink Converter1/LConn1 -- Prismatic Joint (Translational Constraint)/RConn3

== system WECSim_Lib/Frames/Global Reference Frame ==
  note: simu.domainSize
      | waves.waterDepth
  note: Serves as the global reference frame for any WEC-Sim simulation.
      | Has a connection point at (0,0,0), defined at the free surface.
      | Sets up the free surface and ground visualization.
      | Sends the simulation time to a GoTo that can be accesed by other blocks.
  Clock : Clock
  Mean Free Surface : sm_lib/Body Elements/Solid  InertiaType=Custom  Mass=10^20  MassUnits=kg  CenterOfMass=[0 0 0]  CenterOfMassUnits=m  MomentsOfInertia=[10^20 10^20 10^20]  MomentsOfInertiaUnits=kg*m^2  ProductsOfInertia=[0 0 0]  ProductsOfInertiaUnits=kg*m^2  DensityBased=on  Density=1000  DensityUnits=kg/(m^3)  GraphicType=FromGeometry  MarkerShape=Sphere  MarkerSize=10  MarkerSizeUnits=m  GraphicVisPropType=SimpleVisualProperties  GraphicDiffuseColor=[0.0 0.6 0.8]  GraphicSpecularColor=[0.5 0.5 0.5 1.0]  GraphicAmbientColor=[0.15 0.15 0.15 1.0]  GraphicEmissiveColor=[0.0 0.0 0.0 1.0]  GraphicShininess=75  GraphicOpacity=0.3  GeometryShape=GeneralExtrusion  RectangleSize=[1 1]  RectangleSizeUnits=m  BrickDimensions=[1 1 1]  BrickDimensionUnits=m  CylinderRadius=1  CylinderRadiusUnits=m  CylinderLength=1  CylinderLengthUnits=m  SphereRadius=1  SphereRadiusUnits=m  EllipsoidRadii=[1 1 1]  EllipsoidRadiiUnits=m  ExtrusionCrossSection=[simu.domainSize simu.domainSize; -simu.domainSize simu.domainSize; -simu.domainSize -simu.domainSize; simu.domainSize -simu.domainSize]  ExtrusionCrossSectionUnits=m  ExtrusionLength=simu.domainSize/200  ExtrusionLengthUnits=m  PolygonNumSides=3  PolygonOuterRadius=1  PolygonOuterRadiusUnits=m  ExtGeomFileType=STL  ExtGeomFileUnits=m  RevolutionCrossSection=[1 1; 1 -1; 2 -1; 2 1]  RevolutionCrossSectionUnits=m  RevolutionExtent=Full  RevolutionAngle=180  RevolutionAngleUnits=deg  BlockFunction=simmechanics.library.body_elements.solid
  Mechanism Configuration : sm_lib/Utilities/Mechanism Configuration  UniformGravity=Constant  GravityVector=[0 0 0]  GravityUnits=m/s^2  LinearizationDelta=0.001  BlockFunction=simmechanics.library.utilities.mechanism_configuration
  Rigid Transform : sm_lib/Frames and Transforms/Rigid Transform  TranslationMethod=Cartesian  TranslationLengthUnit=m  TranslationStandardAxis=+Z  TranslationStandardOffset=0  TranslationCartesianOffset=[0 0 -waves.waterDepth]  TranslationROffset=0  TranslationROffsetUnits=m  TranslationZOffset=0  TranslationZOffsetUnits=m  TranslationThetaOffset=0  TranslationThetaOffsetUnits=deg  RotationMethod=None  RotationAngleUnits=deg  RotationStandardAxis=+Z  RotationAngle=0  RotationArbitraryAxis=[0 0 1]  FollAlignAxisA=+X  BaseAlignAxisA=+Y  FollAlignAxisB=+Y  BaseAlignAxisB=+Z  RotationMatrix=[1 0 0; 0 1 0; 0 0 1]  BlockFunction=simmechanics.library.frames_transforms.rigid_transform
  Seabed : sm_lib/Body Elements/Solid  InertiaType=Custom  Mass=10^20  MassUnits=kg  CenterOfMass=[0 0 0]  CenterOfMassUnits=m  MomentsOfInertia=[10^20 10^20 10^20]  MomentsOfInertiaUnits=kg*m^2  ProductsOfInertia=[0 0 0]  ProductsOfInertiaUnits=kg*m^2  DensityBased=on  Density=1000  DensityUnits=kg/(m^3)  GraphicType=FromGeometry  MarkerShape=Sphere  MarkerSize=10  MarkerSizeUnits=m  GraphicVisPropType=SimpleVisualProperties  GraphicDiffuseColor=[0.4 0.4 0.0]  GraphicSpecularColor=[0.5 0.5 0.5 1.0]  GraphicAmbientColor=[0.15 0.15 0.15 1.0]  GraphicEmissiveColor=[0.0 0.0 0.0 1.0]  GraphicShininess=75  GraphicOpacity=1  GeometryShape=GeneralExtrusion  RectangleSize=[1 1]  RectangleSizeUnits=m  BrickDimensions=[1 1 1]  BrickDimensionUnits=m  CylinderRadius=1  CylinderRadiusUnits=m  CylinderLength=1  CylinderLengthUnits=m  SphereRadius=1  SphereRadiusUnits=m  EllipsoidRadii=[1 1 1]  EllipsoidRadiiUnits=m  ExtrusionCrossSection=[simu.domainSize simu.domainSize; -simu.domainSize simu.domainSize; -simu.domainSize -simu.domainSize; simu.domainSize -simu.domainSize]  ExtrusionCrossSectionUnits=m  ExtrusionLength=simu.domainSize/100  ExtrusionLengthUnits=m  PolygonNumSides=3  PolygonOuterRadius=1  PolygonOuterRadiusUnits=m  ExtGeomFileType=STL  ExtGeomFileUnits=m  RevolutionCrossSection=[1 1; 1 -1; 2 -1; 2 1]  RevolutionCrossSectionUnits=m  RevolutionExtent=Full  RevolutionAngle=180  RevolutionAngleUnits=deg  BlockFunction=simmechanics.library.body_elements.solid
  Solver Configuration : nesl_utility/Solver Configuration  PhysicalDomain=network_engine_domain  SubClassName=solver  LeftPortType=input  RightPortType=generic  Accelerate=off  Tones=[]  Harmonics=[]  SimulateNoise=off  Profile=off  UseLocalSampling=off  EnableSwitchedLinearOptims=on  FrequencyDomain=off  UseCCode=off  RelTol=0.001  AbsTol=1e-06  MinStep=1e-09  ToWorkspace=off  DoDC=on  ResidualTolerance=1e-9  UseLocalSolver=off  LocalSolverChoice=NE_BACKWARD_EULER_ADVANCER  LocalSolverSampleTime=.001  DoFixedCost=off  MaxNonlinIter=3  MaxModeIter=2  LinearAlgebra=Sparse  DelaysMemoryBudget=1024  AutomaticFiltering=on  FilteringTimeConstant=0.001
  World Frame : sm_lib/Frames and Transforms/World Frame  BlockFunction=simmechanics.library.frames_transforms.world_frame
  Conn : PMIOPort  Port=1  Side=Right
  tag scope: Clock=global
  wires:
  Clock/1 -> [Clock]
  connections:
  Mechanism Configuration/RConn1 -- World Frame/RConn1 -- Solver Configuration/RConn1 -- Conn/RConn1 -- Mean Free Surface/RConn1 -- Rigid Transform/LConn1
  Seabed/RConn1 -- Rigid Transform/RConn1

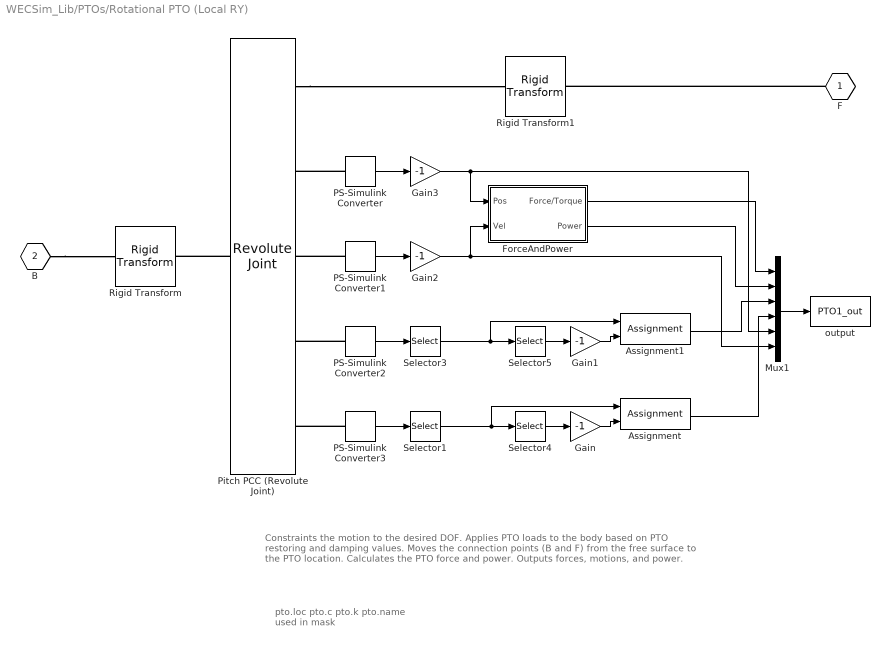
== system WECSim_Lib/PTOs/Rotational PTO (Local RY) ==
  note: pto.loc
      | pto.c
      | pto.k
      | pto.name used in mask
  note: Constraints the motion to the desired DOF.
      | Applies PTO loads to the body based on PTO restoring and damping values.
      | Moves the connection points (B and F) from the free surface to the PTO location.
      | Calculates the PTO force and power.
      | Outputs forces, motions, and power.
  Assignment : Assignment  DiagnosticForDimensions=Warning  Indices=2
  Assignment1 : Assignment  DiagnosticForDimensions=Warning  Indices=2
  ForceAndPower : Subsystem
  Gain{,1..3} (4 alike) : Gain  Gain=-1
  Mux1 : Mux  Inputs=6
  PS-Simulink Converter{,1..3} (4 alike) : nesl_utility/PS-Simulink Converter  PhysicalDomain=network_engine_domain  SubClassName=ps_output  LeftPortType=input  RightPortType=output  PseudoPeriodic=off  Frequencies=[]  Unit=1  AffineConversion=off
  Pitch PCC (Revolute Joint) : sm_lib/Joints/Revolute Joint  SenseConstraintForce=on  SenseConstraintForceX=off  SenseConstraintForceY=off  SenseConstraintForceZ=off  SenseConstraintTorque=on  SenseConstraintTorqueX=off  SenseConstraintTorqueY=off  SenseConstraintTorqueZ=off  SenseTotalForce=off  SenseTotalForceX=off  SenseTotalForceY=off  SenseTotalForceZ=off  SenseTotalTorque=off  SenseTotalTorqueX=off  SenseTotalTorqueY=off  SenseTotalTorqueZ=off  CompositeWrenchDir=BaseOnFollower  CompositeWrenchFrame=BaseFrame  EquilibriumPosition=0  EquilibriumPositionUnits=deg  SpringStiffness=pto.k  SpringStiffnessUnits=N*m/rad  DampingCoefficient=pto.c  DampingCoefficientUnits=N*m/(rad/s)  TorqueActuationMode=NoTorque  MotionActuationMode=ComputedMotion  SensePosition=on  SenseVelocity=on  SenseAcceleration=off  SenseTorqueForce=off  PositionTargetValue=0  PositionTargetValueUnits=deg  PositionTargetSpecify=off  PositionTargetPriority=High  VelocityTargetValue=0  VelocityTargetValueUnits=deg/s  VelocityTargetSpecify=off  VelocityTargetPriority=High  BlockFunction=simmechanics.library.joints.revolute_joint
  Rigid Transform : sm_lib/Frames and Transforms/Rigid Transform  TranslationMethod=Cartesian  TranslationLengthUnit=m  TranslationStandardAxis=+Z  TranslationStandardOffset=0  TranslationCartesianOffset=pto.loc  TranslationROffset=0  TranslationROffsetUnits=m  TranslationZOffset=0  TranslationZOffsetUnits=m  TranslationThetaOffset=0  TranslationThetaOffsetUnits=deg  RotationMethod=StandardAxis  RotationAngleUnits=deg  RotationStandardAxis=+X  RotationAngle=90  RotationArbitraryAxis=[0 0 1]  FollAlignAxisA=+X  BaseAlignAxisA=+Y  FollAlignAxisB=+Y  BaseAlignAxisB=+Z  RotationMatrix=[1 0 0; 0 1 0; 0 0 1]  BlockFunction=simmechanics.library.frames_transforms.rigid_transform
  Rigid Transform1 : sm_lib/Frames and Transforms/Rigid Transform  TranslationMethod=Cartesian  TranslationLengthUnit=m  TranslationStandardAxis=+Z  TranslationStandardOffset=0  TranslationCartesianOffset=pto.loc  TranslationROffset=0  TranslationROffsetUnits=m  TranslationZOffset=0  TranslationZOffsetUnits=m  TranslationThetaOffset=0  TranslationThetaOffsetUnits=deg  RotationMethod=StandardAxis  RotationAngleUnits=deg  RotationStandardAxis=+X  RotationAngle=90  RotationArbitraryAxis=[0 0 1]  FollAlignAxisA=+X  BaseAlignAxisA=+Y  FollAlignAxisB=+Y  BaseAlignAxisB=+Z  RotationMatrix=[1 0 0; 0 1 0; 0 0 1]  BlockFunction=simmechanics.library.frames_transforms.rigid_transform
  Selector1 : Selector  InputPortWidth=3  Indices=[1 3 2]
  Selector3 : Selector  InputPortWidth=3  Indices=[1 3 2]
  Selector4 : Selector  InputPortWidth=3  Indices=[2]
  Selector5 : Selector  InputPortWidth=3  Indices=[2]
  output : ToWorkspace  VariableName=PTO1_out  SaveFormat=Structure With Time  SampleTime=-1
  F : PMIOPort  Port=1  Side=Right
  B : PMIOPort  Port=2  Side=Left
  wires:
  Mux1/1 -> output/1
  ForceAndPower/1(Force/Torque) -> Mux1/1
  ForceAndPower/2(Power) -> Mux1/2
  PS-Simulink Converter2/1 -> Selector3/1
  PS-Simulink Converter3/1 -> Selector1/1
  Selector1/1 -> Assignment/1, Selector4/1
  Selector4/1 -> Gain/1
  Gain/1 -> Assignment/2
  Assignment/1 -> Mux1/4
  Selector3/1 -> Assignment1/1, Selector5/1
  Selector5/1 -> Gain1/1
  Gain1/1 -> Assignment1/2
  Assignment1/1 -> Mux1/3
  PS-Simulink Converter/1 -> Gain3/1
  Gain3/1 -> Mux1/5, ForceAndPower/1(Pos)
  PS-Simulink Converter1/1 -> Gain2/1
  Gain2/1 -> Mux1/6, ForceAndPower/2(Vel)
  connections:
  F/RConn1 -- Rigid Transform1/LConn1
  B/RConn1 -- Rigid Transform/LConn1
  Pitch PCC (Revolute Joint)/RConn1 -- Rigid Transform1/RConn1
  Pitch PCC (Revolute Joint)/LConn1 -- Rigid Transform/RConn1
  PS-Simulink Converter1/LConn1 -- Pitch PCC (Revolute Joint)/RConn3
  PS-Simulink Converter2/LConn1 -- Pitch PCC (Revolute Joint)/RConn4
  PS-Simulink Converter/LConn1 -- Pitch PCC (Revolute Joint)/RConn2
  PS-Simulink Converter3/LConn1 -- Pitch PCC (Revolute Joint)/RConn5

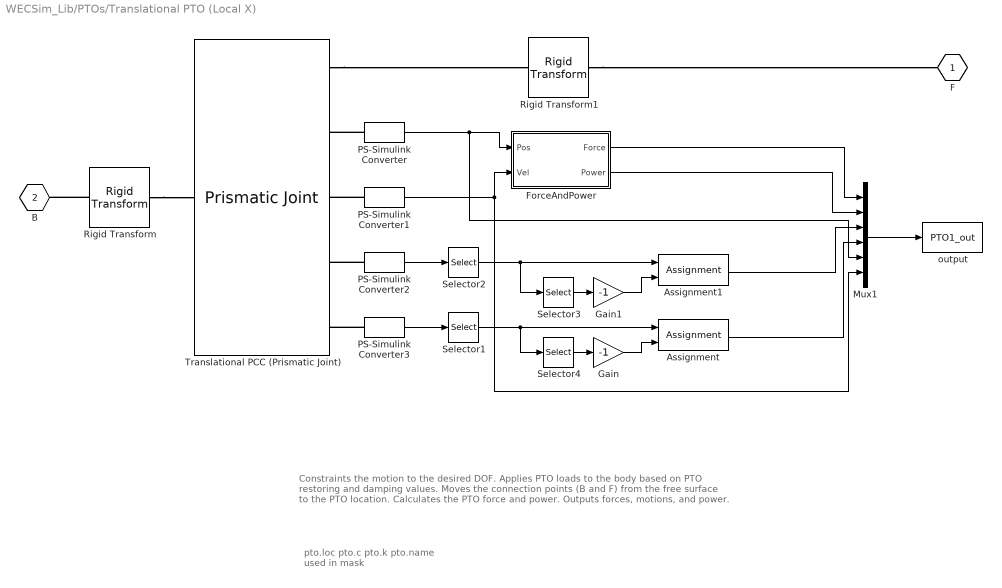
== system WECSim_Lib/PTOs/Translational PTO (Local X) ==
  note: pto.loc
      | pto.c
      | pto.k
      | pto.name used in mask
  note: Constraints the motion to the desired DOF.
      | Applies PTO loads to the body based on PTO restoring and damping values.
      | Moves the connection points (B and F) from the free surface to the PTO location.
      | Calculates the PTO force and power.
      | Outputs forces, motions, and power.
  Assignment : Assignment  DiagnosticForDimensions=Warning  Indices=3
  Assignment1 : Assignment  DiagnosticForDimensions=Warning  Indices=3
  ForceAndPower : Subsystem
  Gain : Gain  Gain=-1
  Gain1 : Gain  Gain=-1
  Mux1 : Mux  Inputs=6
  PS-Simulink Converter{,1..3} (4 alike) : nesl_utility/PS-Simulink Converter  PhysicalDomain=network_engine_domain  SubClassName=ps_output  LeftPortType=input  RightPortType=output  PseudoPeriodic=off  Frequencies=[]  Unit=1  AffineConversion=off
  Rigid Transform : sm_lib/Frames and Transforms/Rigid Transform  TranslationMethod=Cartesian  TranslationLengthUnit=m  TranslationStandardAxis=+Z  TranslationStandardOffset=0  TranslationCartesianOffset=pto.loc  TranslationROffset=0  TranslationROffsetUnits=m  TranslationZOffset=0  TranslationZOffsetUnits=m  TranslationThetaOffset=0  TranslationThetaOffsetUnits=deg  RotationMethod=StandardAxis  RotationAngleUnits=deg  RotationStandardAxis=+Y  RotationAngle=90  RotationArbitraryAxis=[0 0 1]  FollAlignAxisA=+X  BaseAlignAxisA=+Y  FollAlignAxisB=+Y  BaseAlignAxisB=+Z  RotationMatrix=[1 0 0; 0 1 0; 0 0 1]  BlockFunction=simmechanics.library.frames_transforms.rigid_transform
  Rigid Transform1 : sm_lib/Frames and Transforms/Rigid Transform  TranslationMethod=Cartesian  TranslationLengthUnit=m  TranslationStandardAxis=+Z  TranslationStandardOffset=0  TranslationCartesianOffset=pto.loc  TranslationROffset=0  TranslationROffsetUnits=m  TranslationZOffset=0  TranslationZOffsetUnits=m  TranslationThetaOffset=0  TranslationThetaOffsetUnits=deg  RotationMethod=StandardAxis  RotationAngleUnits=deg  RotationStandardAxis=+Y  RotationAngle=90  RotationArbitraryAxis=[0 0 1]  FollAlignAxisA=+X  BaseAlignAxisA=+Y  FollAlignAxisB=+Y  BaseAlignAxisB=+Z  RotationMatrix=[1 0 0; 0 1 0; 0 0 1]  BlockFunction=simmechanics.library.frames_transforms.rigid_transform
  Selector1 : Selector  InputPortWidth=3  Indices=[3 2 1]
  Selector2 : Selector  InputPortWidth=3  Indices=[3 2 1]
  Selector3 : Selector  InputPortWidth=3  Indices=[3]
  Selector4 : Selector  InputPortWidth=3  Indices=[3]
  Translational PCC (Prismatic Joint) : sm_lib/Joints/Prismatic Joint  SenseConstraintForce=on  SenseConstraintForceX=off  SenseConstraintForceY=off  SenseConstraintForceZ=off  SenseConstraintTorque=on  SenseConstraintTorqueX=off  SenseConstraintTorqueY=off  SenseConstraintTorqueZ=off  SenseTotalForce=off  SenseTotalForceX=off  SenseTotalForceY=off  SenseTotalForceZ=off  SenseTotalTorque=off  SenseTotalTorqueX=off  SenseTotalTorqueY=off  SenseTotalTorqueZ=off  CompositeWrenchDir=BaseOnFollower  CompositeWrenchFrame=BaseFrame  EquilibriumPosition=0  EquilibriumPositionUnits=m  SpringStiffness=pto.k  SpringStiffnessUnits=N/m  DampingCoefficient=pto.c  DampingCoefficientUnits=N/(m/s)  TorqueActuationMode=NoTorque  MotionActuationMode=ComputedMotion  SensePosition=on  SenseVelocity=on  SenseAcceleration=off  SenseTorqueForce=off  PositionTargetValue=0  PositionTargetValueUnits=m  PositionTargetSpecify=off  PositionTargetPriority=High  VelocityTargetValue=0  VelocityTargetValueUnits=m/s  VelocityTargetSpecify=off  VelocityTargetPriority=High  BlockFunction=simmechanics.library.joints.prismatic_joint
  output : ToWorkspace  VariableName=PTO1_out  SaveFormat=Structure With Time  SampleTime=-1
  F : PMIOPort  Port=1  Side=Left
  B : PMIOPort  Port=2  Side=Right
  wires:
  PS-Simulink Converter1/1 -> Mux1/6, ForceAndPower/2(Vel)
  Mux1/1 -> output/1
  ForceAndPower/1(Force) -> Mux1/1
  ForceAndPower/2(Power) -> Mux1/2
  PS-Simulink Converter/1 -> Mux1/5, ForceAndPower/1(Pos)
  Selector1/1 -> Selector4/1, Assignment/1
  Selector4/1 -> Gain/1
  Gain/1 -> Assignment/2
  Selector2/1 -> Selector3/1, Assignment1/1
  Selector3/1 -> Gain1/1
  Gain1/1 -> Assignment1/2
  PS-Simulink Converter3/1 -> Selector1/1
  PS-Simulink Converter2/1 -> Selector2/1
  Assignment/1 -> Mux1/4
  Assignment1/1 -> Mux1/3
  connections:
  Rigid Transform/LConn1 -- B/RConn1
  Rigid Transform/RConn1 -- Translational PCC (Prismatic Joint)/LConn1
  Translational PCC (Prismatic Joint)/RConn1 -- Rigid Transform1/RConn1
  Rigid Transform1/LConn1 -- F/RConn1
  PS-Simulink Converter/LConn1 -- Translational PCC (Prismatic Joint)/RConn2
  PS-Simulink Converter1/LConn1 -- Translational PCC (Prismatic Joint)/RConn3
  PS-Simulink Converter2/LConn1 -- Translational PCC (Prismatic Joint)/RConn4
  PS-Simulink Converter3/LConn1 -- Translational PCC (Prismatic Joint)/RConn5
